simulink model "pfb_fir_generic_test_sim3"  (R2012b)
settings: Solver=VariableStepDiscrete  StartTime=0.0  StopTime=10.0  RelTol=1e-3
model workspace (MAT data in the model file):
  synci = [0 1 2 3 4 5 6 7 8 9 10 11 ... (589826 elements, 294913x2)]
  din0 = [0 1 2 3 4 5 6 7 8 9 10 11 ... (73730 elements, 36865x2)]
  din1 = [0 1 2 3 4 5 6 7 8 9 10 11 ... (73730 elements, 36865x2)]
  din2 = [0 1 2 3 4 5 6 7 8 9 10 11 ... (73730 elements, 36865x2)]
  din3 = [0 1 2 3 4 5 6 7 8 9 10 11 ... (73730 elements, 36865x2)]
  din4 = [0 1 2 3 4 5 6 7 8 9 10 11 ... (73730 elements, 36865x2)]
  din5 = [0 1 2 3 4 5 6 7 8 9 10 11 ... (73730 elements, 36865x2)]
  din6 = [0 1 2 3 4 5 6 7 8 9 10 11 ... (73730 elements, 36865x2)]
  din7 = [0 1 2 3 4 5 6 7 8 9 10 11 ... (73730 elements, 36865x2)]
libraries: xbsIndex_r4 x5585, casper_library_delays x1
(part 21 of 25)

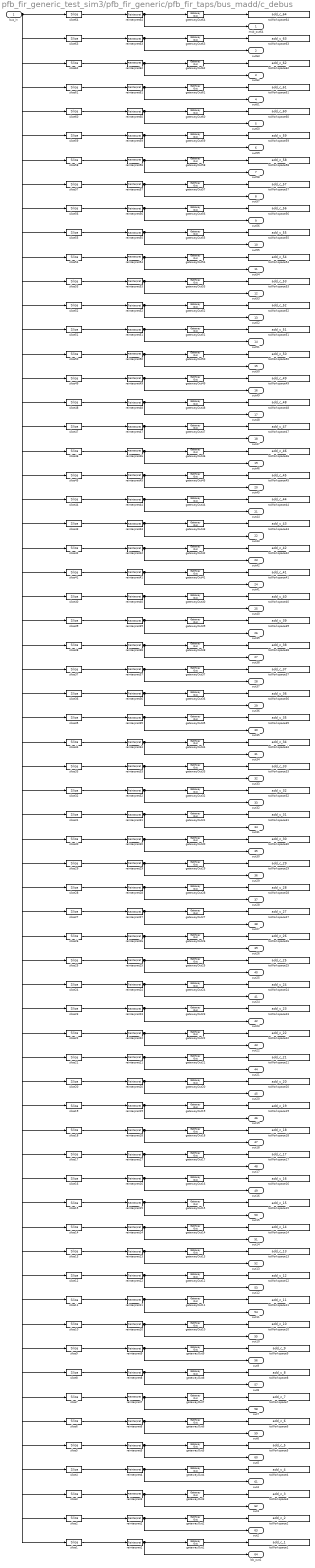
== system pfb_fir_generic_test_sim3/pfb_fir_generic/pfb_fir_taps/bus_madd/c_debus ==
  bus_in : Inport
  gatewayOut{1..64} (64 alike) : xbsIndex_r4/Gateway Out  inherit_from_input=off  hdl_port=off  timing_constraint=None  locs_specified=off  LOCs={}  UseAsDAC=off  DACChannel='1'  block_type=gatewayout
  reinterpret{1..64} (64 alike) : xbsIndex_r4/Reinterpret  force_arith_type=on  arith_type="Signed  (2's comp)"  force_bin_pt=on  bin_pt=26  block_type=reinterpret
  slice1 : xbsIndex_r4/Slice  nbits=30  boolean_output=off  mode=Upper Bit Location + Width  bit1=-1810  base1=MSB of Input  bit0=0  base0=LSB of Input  dbl_ovrd=off  block_type=slice
  slice10 : xbsIndex_r4/Slice  nbits=30  boolean_output=off  mode=Upper Bit Location + Width  bit1=-1540  base1=MSB of Input  bit0=0  base0=LSB of Input  dbl_ovrd=off  block_type=slice
  slice11 : xbsIndex_r4/Slice  nbits=30  boolean_output=off  mode=Upper Bit Location + Width  bit1=-1510  base1=MSB of Input  bit0=0  base0=LSB of Input  dbl_ovrd=off  block_type=slice
  slice12 : xbsIndex_r4/Slice  nbits=30  boolean_output=off  mode=Upper Bit Location + Width  bit1=-1480  base1=MSB of Input  bit0=0  base0=LSB of Input  dbl_ovrd=off  block_type=slice
  slice13 : xbsIndex_r4/Slice  nbits=30  boolean_output=off  mode=Upper Bit Location + Width  bit1=-1450  base1=MSB of Input  bit0=0  base0=LSB of Input  dbl_ovrd=off  block_type=slice
  slice14 : xbsIndex_r4/Slice  nbits=30  boolean_output=off  mode=Upper Bit Location + Width  bit1=-1420  base1=MSB of Input  bit0=0  base0=LSB of Input  dbl_ovrd=off  block_type=slice
  slice15 : xbsIndex_r4/Slice  nbits=30  boolean_output=off  mode=Upper Bit Location + Width  bit1=-1390  base1=MSB of Input  bit0=0  base0=LSB of Input  dbl_ovrd=off  block_type=slice
  slice16 : xbsIndex_r4/Slice  nbits=30  boolean_output=off  mode=Upper Bit Location + Width  bit1=-1360  base1=MSB of Input  bit0=0  base0=LSB of Input  dbl_ovrd=off  block_type=slice
  slice17 : xbsIndex_r4/Slice  nbits=29  boolean_output=off  mode=Upper Bit Location + Width  bit1=-1331  base1=MSB of Input  bit0=0  base0=LSB of Input  dbl_ovrd=off  block_type=slice
  slice18 : xbsIndex_r4/Slice  nbits=29  boolean_output=off  mode=Upper Bit Location + Width  bit1=-1302  base1=MSB of Input  bit0=0  base0=LSB of Input  dbl_ovrd=off  block_type=slice
  slice19 : xbsIndex_r4/Slice  nbits=29  boolean_output=off  mode=Upper Bit Location + Width  bit1=-1273  base1=MSB of Input  bit0=0  base0=LSB of Input  dbl_ovrd=off  block_type=slice
  slice2 : xbsIndex_r4/Slice  nbits=30  boolean_output=off  mode=Upper Bit Location + Width  bit1=-1780  base1=MSB of Input  bit0=0  base0=LSB of Input  dbl_ovrd=off  block_type=slice
  slice20 : xbsIndex_r4/Slice  nbits=29  boolean_output=off  mode=Upper Bit Location + Width  bit1=-1244  base1=MSB of Input  bit0=0  base0=LSB of Input  dbl_ovrd=off  block_type=slice
  slice21 : xbsIndex_r4/Slice  nbits=29  boolean_output=off  mode=Upper Bit Location + Width  bit1=-1215  base1=MSB of Input  bit0=0  base0=LSB of Input  dbl_ovrd=off  block_type=slice
  slice22 : xbsIndex_r4/Slice  nbits=29  boolean_output=off  mode=Upper Bit Location + Width  bit1=-1186  base1=MSB of Input  bit0=0  base0=LSB of Input  dbl_ovrd=off  block_type=slice
  slice23 : xbsIndex_r4/Slice  nbits=29  boolean_output=off  mode=Upper Bit Location + Width  bit1=-1157  base1=MSB of Input  bit0=0  base0=LSB of Input  dbl_ovrd=off  block_type=slice
  slice24 : xbsIndex_r4/Slice  nbits=29  boolean_output=off  mode=Upper Bit Location + Width  bit1=-1128  base1=MSB of Input  bit0=0  base0=LSB of Input  dbl_ovrd=off  block_type=slice
  slice25 : xbsIndex_r4/Slice  nbits=29  boolean_output=off  mode=Upper Bit Location + Width  bit1=-1099  base1=MSB of Input  bit0=0  base0=LSB of Input  dbl_ovrd=off  block_type=slice
  slice26 : xbsIndex_r4/Slice  nbits=29  boolean_output=off  mode=Upper Bit Location + Width  bit1=-1070  base1=MSB of Input  bit0=0  base0=LSB of Input  dbl_ovrd=off  block_type=slice
  slice27 : xbsIndex_r4/Slice  nbits=29  boolean_output=off  mode=Upper Bit Location + Width  bit1=-1041  base1=MSB of Input  bit0=0  base0=LSB of Input  dbl_ovrd=off  block_type=slice
  slice28 : xbsIndex_r4/Slice  nbits=29  boolean_output=off  mode=Upper Bit Location + Width  bit1=-1012  base1=MSB of Input  bit0=0  base0=LSB of Input  dbl_ovrd=off  block_type=slice
  slice29 : xbsIndex_r4/Slice  nbits=29  boolean_output=off  mode=Upper Bit Location + Width  bit1=-983  base1=MSB of Input  bit0=0  base0=LSB of Input  dbl_ovrd=off  block_type=slice
  slice3 : xbsIndex_r4/Slice  nbits=30  boolean_output=off  mode=Upper Bit Location + Width  bit1=-1750  base1=MSB of Input  bit0=0  base0=LSB of Input  dbl_ovrd=off  block_type=slice
  slice30 : xbsIndex_r4/Slice  nbits=29  boolean_output=off  mode=Upper Bit Location + Width  bit1=-954  base1=MSB of Input  bit0=0  base0=LSB of Input  dbl_ovrd=off  block_type=slice
  slice31 : xbsIndex_r4/Slice  nbits=29  boolean_output=off  mode=Upper Bit Location + Width  bit1=-925  base1=MSB of Input  bit0=0  base0=LSB of Input  dbl_ovrd=off  block_type=slice
  slice32 : xbsIndex_r4/Slice  nbits=29  boolean_output=off  mode=Upper Bit Location + Width  bit1=-896  base1=MSB of Input  bit0=0  base0=LSB of Input  dbl_ovrd=off  block_type=slice
  slice33 : xbsIndex_r4/Slice  nbits=28  boolean_output=off  mode=Upper Bit Location + Width  bit1=-868  base1=MSB of Input  bit0=0  base0=LSB of Input  dbl_ovrd=off  block_type=slice
  slice34 : xbsIndex_r4/Slice  nbits=28  boolean_output=off  mode=Upper Bit Location + Width  bit1=-840  base1=MSB of Input  bit0=0  base0=LSB of Input  dbl_ovrd=off  block_type=slice
  slice35 : xbsIndex_r4/Slice  nbits=28  boolean_output=off  mode=Upper Bit Location + Width  bit1=-812  base1=MSB of Input  bit0=0  base0=LSB of Input  dbl_ovrd=off  block_type=slice
  slice36 : xbsIndex_r4/Slice  nbits=28  boolean_output=off  mode=Upper Bit Location + Width  bit1=-784  base1=MSB of Input  bit0=0  base0=LSB of Input  dbl_ovrd=off  block_type=slice
  slice37 : xbsIndex_r4/Slice  nbits=28  boolean_output=off  mode=Upper Bit Location + Width  bit1=-756  base1=MSB of Input  bit0=0  base0=LSB of Input  dbl_ovrd=off  block_type=slice
  slice38 : xbsIndex_r4/Slice  nbits=28  boolean_output=off  mode=Upper Bit Location + Width  bit1=-728  base1=MSB of Input  bit0=0  base0=LSB of Input  dbl_ovrd=off  block_type=slice
  slice39 : xbsIndex_r4/Slice  nbits=28  boolean_output=off  mode=Upper Bit Location + Width  bit1=-700  base1=MSB of Input  bit0=0  base0=LSB of Input  dbl_ovrd=off  block_type=slice
  slice4 : xbsIndex_r4/Slice  nbits=30  boolean_output=off  mode=Upper Bit Location + Width  bit1=-1720  base1=MSB of Input  bit0=0  base0=LSB of Input  dbl_ovrd=off  block_type=slice
  slice40 : xbsIndex_r4/Slice  nbits=28  boolean_output=off  mode=Upper Bit Location + Width  bit1=-672  base1=MSB of Input  bit0=0  base0=LSB of Input  dbl_ovrd=off  block_type=slice
  slice41 : xbsIndex_r4/Slice  nbits=28  boolean_output=off  mode=Upper Bit Location + Width  bit1=-644  base1=MSB of Input  bit0=0  base0=LSB of Input  dbl_ovrd=off  block_type=slice
  slice42 : xbsIndex_r4/Slice  nbits=28  boolean_output=off  mode=Upper Bit Location + Width  bit1=-616  base1=MSB of Input  bit0=0  base0=LSB of Input  dbl_ovrd=off  block_type=slice
  slice43 : xbsIndex_r4/Slice  nbits=28  boolean_output=off  mode=Upper Bit Location + Width  bit1=-588  base1=MSB of Input  bit0=0  base0=LSB of Input  dbl_ovrd=off  block_type=slice
  slice44 : xbsIndex_r4/Slice  nbits=28  boolean_output=off  mode=Upper Bit Location + Width  bit1=-560  base1=MSB of Input  bit0=0  base0=LSB of Input  dbl_ovrd=off  block_type=slice
  slice45 : xbsIndex_r4/Slice  nbits=28  boolean_output=off  mode=Upper Bit Location + Width  bit1=-532  base1=MSB of Input  bit0=0  base0=LSB of Input  dbl_ovrd=off  block_type=slice
  slice46 : xbsIndex_r4/Slice  nbits=28  boolean_output=off  mode=Upper Bit Location + Width  bit1=-504  base1=MSB of Input  bit0=0  base0=LSB of Input  dbl_ovrd=off  block_type=slice
  slice47 : xbsIndex_r4/Slice  nbits=28  boolean_output=off  mode=Upper Bit Location + Width  bit1=-476  base1=MSB of Input  bit0=0  base0=LSB of Input  dbl_ovrd=off  block_type=slice
  slice48 : xbsIndex_r4/Slice  nbits=28  boolean_output=off  mode=Upper Bit Location + Width  bit1=-448  base1=MSB of Input  bit0=0  base0=LSB of Input  dbl_ovrd=off  block_type=slice
  slice49 : xbsIndex_r4/Slice  nbits=28  boolean_output=off  mode=Upper Bit Location + Width  bit1=-420  base1=MSB of Input  bit0=0  base0=LSB of Input  dbl_ovrd=off  block_type=slice
  slice5 : xbsIndex_r4/Slice  nbits=30  boolean_output=off  mode=Upper Bit Location + Width  bit1=-1690  base1=MSB of Input  bit0=0  base0=LSB of Input  dbl_ovrd=off  block_type=slice
  slice50 : xbsIndex_r4/Slice  nbits=28  boolean_output=off  mode=Upper Bit Location + Width  bit1=-392  base1=MSB of Input  bit0=0  base0=LSB of Input  dbl_ovrd=off  block_type=slice
  slice51 : xbsIndex_r4/Slice  nbits=28  boolean_output=off  mode=Upper Bit Location + Width  bit1=-364  base1=MSB of Input  bit0=0  base0=LSB of Input  dbl_ovrd=off  block_type=slice
  slice52 : xbsIndex_r4/Slice  nbits=28  boolean_output=off  mode=Upper Bit Location + Width  bit1=-336  base1=MSB of Input  bit0=0  base0=LSB of Input  dbl_ovrd=off  block_type=slice
  slice53 : xbsIndex_r4/Slice  nbits=28  boolean_output=off  mode=Upper Bit Location + Width  bit1=-308  base1=MSB of Input  bit0=0  base0=LSB of Input  dbl_ovrd=off  block_type=slice
  slice54 : xbsIndex_r4/Slice  nbits=28  boolean_output=off  mode=Upper Bit Location + Width  bit1=-280  base1=MSB of Input  bit0=0  base0=LSB of Input  dbl_ovrd=off  block_type=slice
  slice55 : xbsIndex_r4/Slice  nbits=28  boolean_output=off  mode=Upper Bit Location + Width  bit1=-252  base1=MSB of Input  bit0=0  base0=LSB of Input  dbl_ovrd=off  block_type=slice
  slice56 : xbsIndex_r4/Slice  nbits=28  boolean_output=off  mode=Upper Bit Location + Width  bit1=-224  base1=MSB of Input  bit0=0  base0=LSB of Input  dbl_ovrd=off  block_type=slice
  slice57 : xbsIndex_r4/Slice  nbits=28  boolean_output=off  mode=Upper Bit Location + Width  bit1=-196  base1=MSB of Input  bit0=0  base0=LSB of Input  dbl_ovrd=off  block_type=slice
  slice58 : xbsIndex_r4/Slice  nbits=28  boolean_output=off  mode=Upper Bit Location + Width  bit1=-168  base1=MSB of Input  bit0=0  base0=LSB of Input  dbl_ovrd=off  block_type=slice
  slice59 : xbsIndex_r4/Slice  nbits=28  boolean_output=off  mode=Upper Bit Location + Width  bit1=-140  base1=MSB of Input  bit0=0  base0=LSB of Input  dbl_ovrd=off  block_type=slice
  slice6 : xbsIndex_r4/Slice  nbits=30  boolean_output=off  mode=Upper Bit Location + Width  bit1=-1660  base1=MSB of Input  bit0=0  base0=LSB of Input  dbl_ovrd=off  block_type=slice
  slice60 : xbsIndex_r4/Slice  nbits=28  boolean_output=off  mode=Upper Bit Location + Width  bit1=-112  base1=MSB of Input  bit0=0  base0=LSB of Input  dbl_ovrd=off  block_type=slice
  slice61 : xbsIndex_r4/Slice  nbits=28  boolean_output=off  mode=Upper Bit Location + Width  bit1=-84  base1=MSB of Input  bit0=0  base0=LSB of Input  dbl_ovrd=off  block_type=slice
  slice62 : xbsIndex_r4/Slice  nbits=28  boolean_output=off  mode=Upper Bit Location + Width  bit1=-56  base1=MSB of Input  bit0=0  base0=LSB of Input  dbl_ovrd=off  block_type=slice
  slice63 : xbsIndex_r4/Slice  nbits=28  boolean_output=off  mode=Upper Bit Location + Width  bit1=-28  base1=MSB of Input  bit0=0  base0=LSB of Input  dbl_ovrd=off  block_type=slice
  slice64 : xbsIndex_r4/Slice  nbits=28  boolean_output=off  mode=Upper Bit Location + Width  bit1=0  base1=MSB of Input  bit0=0  base0=LSB of Input  dbl_ovrd=off  block_type=slice
  slice7 : xbsIndex_r4/Slice  nbits=30  boolean_output=off  mode=Upper Bit Location + Width  bit1=-1630  base1=MSB of Input  bit0=0  base0=LSB of Input  dbl_ovrd=off  block_type=slice
  slice8 : xbsIndex_r4/Slice  nbits=30  boolean_output=off  mode=Upper Bit Location + Width  bit1=-1600  base1=MSB of Input  bit0=0  base0=LSB of Input  dbl_ovrd=off  block_type=slice
  slice9 : xbsIndex_r4/Slice  nbits=30  boolean_output=off  mode=Upper Bit Location + Width  bit1=-1570  base1=MSB of Input  bit0=0  base0=LSB of Input  dbl_ovrd=off  block_type=slice
  toWorkspace1 : ToWorkspace  VariableName=add_c_1  SampleTime=-1  SaveFormat=Structure With Time
  toWorkspace10 : ToWorkspace  VariableName=add_c_10  SampleTime=-1  SaveFormat=Structure With Time
  toWorkspace11 : ToWorkspace  VariableName=add_c_11  SampleTime=-1  SaveFormat=Structure With Time
  toWorkspace12 : ToWorkspace  VariableName=add_c_12  SampleTime=-1  SaveFormat=Structure With Time
  toWorkspace13 : ToWorkspace  VariableName=add_c_13  SampleTime=-1  SaveFormat=Structure With Time
  toWorkspace14 : ToWorkspace  VariableName=add_c_14  SampleTime=-1  SaveFormat=Structure With Time
  toWorkspace15 : ToWorkspace  VariableName=add_c_15  SampleTime=-1  SaveFormat=Structure With Time
  toWorkspace16 : ToWorkspace  VariableName=add_c_16  SampleTime=-1  SaveFormat=Structure With Time
  toWorkspace17 : ToWorkspace  VariableName=add_c_17  SampleTime=-1  SaveFormat=Structure With Time
  toWorkspace18 : ToWorkspace  VariableName=add_c_18  SampleTime=-1  SaveFormat=Structure With Time
  toWorkspace19 : ToWorkspace  VariableName=add_c_19  SampleTime=-1  SaveFormat=Structure With Time
  toWorkspace2 : ToWorkspace  VariableName=add_c_2  SampleTime=-1  SaveFormat=Structure With Time
  toWorkspace20 : ToWorkspace  VariableName=add_c_20  SampleTime=-1  SaveFormat=Structure With Time
  toWorkspace21 : ToWorkspace  VariableName=add_c_21  SampleTime=-1  SaveFormat=Structure With Time
  toWorkspace22 : ToWorkspace  VariableName=add_c_22  SampleTime=-1  SaveFormat=Structure With Time
  toWorkspace23 : ToWorkspace  VariableName=add_c_23  SampleTime=-1  SaveFormat=Structure With Time
  toWorkspace24 : ToWorkspace  VariableName=add_c_24  SampleTime=-1  SaveFormat=Structure With Time
  toWorkspace25 : ToWorkspace  VariableName=add_c_25  SampleTime=-1  SaveFormat=Structure With Time
  toWorkspace26 : ToWorkspace  VariableName=add_c_26  SampleTime=-1  SaveFormat=Structure With Time
  toWorkspace27 : ToWorkspace  VariableName=add_c_27  SampleTime=-1  SaveFormat=Structure With Time
  toWorkspace28 : ToWorkspace  VariableName=add_c_28  SampleTime=-1  SaveFormat=Structure With Time
  toWorkspace29 : ToWorkspace  VariableName=add_c_29  SampleTime=-1  SaveFormat=Structure With Time
  toWorkspace3 : ToWorkspace  VariableName=add_c_3  SampleTime=-1  SaveFormat=Structure With Time
  toWorkspace30 : ToWorkspace  VariableName=add_c_30  SampleTime=-1  SaveFormat=Structure With Time
  toWorkspace31 : ToWorkspace  VariableName=add_c_31  SampleTime=-1  SaveFormat=Structure With Time
  toWorkspace32 : ToWorkspace  VariableName=add_c_32  SampleTime=-1  SaveFormat=Structure With Time
  toWorkspace33 : ToWorkspace  VariableName=add_c_33  SampleTime=-1  SaveFormat=Structure With Time
  toWorkspace34 : ToWorkspace  VariableName=add_c_34  SampleTime=-1  SaveFormat=Structure With Time
  toWorkspace35 : ToWorkspace  VariableName=add_c_35  SampleTime=-1  SaveFormat=Structure With Time
  toWorkspace36 : ToWorkspace  VariableName=add_c_36  SampleTime=-1  SaveFormat=Structure With Time
  toWorkspace37 : ToWorkspace  VariableName=add_c_37  SampleTime=-1  SaveFormat=Structure With Time
  toWorkspace38 : ToWorkspace  VariableName=add_c_38  SampleTime=-1  SaveFormat=Structure With Time
  toWorkspace39 : ToWorkspace  VariableName=add_c_39  SampleTime=-1  SaveFormat=Structure With Time
  toWorkspace4 : ToWorkspace  VariableName=add_c_4  SampleTime=-1  SaveFormat=Structure With Time
  toWorkspace40 : ToWorkspace  VariableName=add_c_40  SampleTime=-1  SaveFormat=Structure With Time
  toWorkspace41 : ToWorkspace  VariableName=add_c_41  SampleTime=-1  SaveFormat=Structure With Time
  toWorkspace42 : ToWorkspace  VariableName=add_c_42  SampleTime=-1  SaveFormat=Structure With Time
  toWorkspace43 : ToWorkspace  VariableName=add_c_43  SampleTime=-1  SaveFormat=Structure With Time
  toWorkspace44 : ToWorkspace  VariableName=add_c_44  SampleTime=-1  SaveFormat=Structure With Time
  toWorkspace45 : ToWorkspace  VariableName=add_c_45  SampleTime=-1  SaveFormat=Structure With Time
  toWorkspace46 : ToWorkspace  VariableName=add_c_46  SampleTime=-1  SaveFormat=Structure With Time
  toWorkspace47 : ToWorkspace  VariableName=add_c_47  SampleTime=-1  SaveFormat=Structure With Time
  toWorkspace48 : ToWorkspace  VariableName=add_c_48  SampleTime=-1  SaveFormat=Structure With Time
  toWorkspace49 : ToWorkspace  VariableName=add_c_49  SampleTime=-1  SaveFormat=Structure With Time
  toWorkspace5 : ToWorkspace  VariableName=add_c_5  SampleTime=-1  SaveFormat=Structure With Time
  toWorkspace50 : ToWorkspace  VariableName=add_c_50  SampleTime=-1  SaveFormat=Structure With Time
  toWorkspace51 : ToWorkspace  VariableName=add_c_51  SampleTime=-1  SaveFormat=Structure With Time
  toWorkspace52 : ToWorkspace  VariableName=add_c_52  SampleTime=-1  SaveFormat=Structure With Time
  toWorkspace53 : ToWorkspace  VariableName=add_c_53  SampleTime=-1  SaveFormat=Structure With Time
  toWorkspace54 : ToWorkspace  VariableName=add_c_54  SampleTime=-1  SaveFormat=Structure With Time
  toWorkspace55 : ToWorkspace  VariableName=add_c_55  SampleTime=-1  SaveFormat=Structure With Time
  toWorkspace56 : ToWorkspace  VariableName=add_c_56  SampleTime=-1  SaveFormat=Structure With Time
  toWorkspace57 : ToWorkspace  VariableName=add_c_57  SampleTime=-1  SaveFormat=Structure With Time
  toWorkspace58 : ToWorkspace  VariableName=add_c_58  SampleTime=-1  SaveFormat=Structure With Time
  toWorkspace59 : ToWorkspace  VariableName=add_c_59  SampleTime=-1  SaveFormat=Structure With Time
  toWorkspace6 : ToWorkspace  VariableName=add_c_6  SampleTime=-1  SaveFormat=Structure With Time
  toWorkspace60 : ToWorkspace  VariableName=add_c_60  SampleTime=-1  SaveFormat=Structure With Time
  toWorkspace61 : ToWorkspace  VariableName=add_c_61  SampleTime=-1  SaveFormat=Structure With Time
  toWorkspace62 : ToWorkspace  VariableName=add_c_62  SampleTime=-1  SaveFormat=Structure With Time
  toWorkspace63 : ToWorkspace  VariableName=add_c_63  SampleTime=-1  SaveFormat=Structure With Time
  toWorkspace64 : ToWorkspace  VariableName=add_c_64  SampleTime=-1  SaveFormat=Structure With Time
  toWorkspace7 : ToWorkspace  VariableName=add_c_7  SampleTime=-1  SaveFormat=Structure With Time
  toWorkspace8 : ToWorkspace  VariableName=add_c_8  SampleTime=-1  SaveFormat=Structure With Time
  toWorkspace9 : ToWorkspace  VariableName=add_c_9  SampleTime=-1  SaveFormat=Structure With Time
  msb_out64 : Outport
  out63 : Outport  Port=2
  out62 : Outport  Port=3
  out61 : Outport  Port=4
  out60 : Outport  Port=5
  out59 : Outport  Port=6
  out58 : Outport  Port=7
  out57 : Outport  Port=8
  out56 : Outport  Port=9
  out55 : Outport  Port=10
  out54 : Outport  Port=11
  out53 : Outport  Port=12
  out52 : Outport  Port=13
  out51 : Outport  Port=14
  out50 : Outport  Port=15
  out49 : Outport  Port=16
  out48 : Outport  Port=17
  out47 : Outport  Port=18
  out46 : Outport  Port=19
  out45 : Outport  Port=20
  out44 : Outport  Port=21
  out43 : Outport  Port=22
  out42 : Outport  Port=23
  out41 : Outport  Port=24
  out40 : Outport  Port=25
  out39 : Outport  Port=26
  out38 : Outport  Port=27
  out37 : Outport  Port=28
  out36 : Outport  Port=29
  out35 : Outport  Port=30
  out34 : Outport  Port=31
  out33 : Outport  Port=32
  out32 : Outport  Port=33
  out31 : Outport  Port=34
  out30 : Outport  Port=35
  out29 : Outport  Port=36
  out28 : Outport  Port=37
  out27 : Outport  Port=38
  out26 : Outport  Port=39
  out25 : Outport  Port=40
  out24 : Outport  Port=41
  out23 : Outport  Port=42
  out22 : Outport  Port=43
  out21 : Outport  Port=44
  out20 : Outport  Port=45
  out19 : Outport  Port=46
  out18 : Outport  Port=47
  out17 : Outport  Port=48
  out16 : Outport  Port=49
  out15 : Outport  Port=50
  out14 : Outport  Port=51
  out13 : Outport  Port=52
  out12 : Outport  Port=53
  out11 : Outport  Port=54
  out10 : Outport  Port=55
  out9 : Outport  Port=56
  out8 : Outport  Port=57
  out7 : Outport  Port=58
  out6 : Outport  Port=59
  out5 : Outport  Port=60
  out4 : Outport  Port=61
  out3 : Outport  Port=62
  out2 : Outport  Port=63
  lsb_out1 : Outport  Port=64
  wires:
  bus_in/1 -> slice64/1, slice63/1, slice62/1, slice61/1, slice60/1, slice59/1, slice58/1, slice57/1, slice56/1, slice55/1, slice54/1, slice53/1, slice52/1, slice51/1, slice50/1, slice49/1, slice48/1, slice47/1, slice46/1, slice45/1, slice44/1, slice43/1, slice42/1, slice41/1, slice40/1, slice39/1, slice38/1, slice37/1, slice36/1, slice35/1, slice34/1, slice33/1, slice32/1, slice31/1, slice30/1, slice29/1, slice28/1, slice27/1, slice26/1, slice25/1, slice24/1, slice23/1, slice22/1, slice21/1, slice20/1, slice19/1, slice18/1, slice17/1, slice16/1, slice15/1, slice14/1, slice13/1, slice12/1, slice11/1, slice10/1, slice9/1, slice8/1, slice7/1, slice6/1, slice5/1, slice4/1, slice3/1, slice2/1, slice1/1
  slice64/1 -> reinterpret64/1
  reinterpret64/1 -> gatewayOut64/1, msb_out64/1
  gatewayOut64/1 -> toWorkspace64/1
  slice63/1 -> reinterpret63/1
  reinterpret63/1 -> gatewayOut63/1, out63/1
  gatewayOut63/1 -> toWorkspace63/1
  slice62/1 -> reinterpret62/1
  reinterpret62/1 -> gatewayOut62/1, out62/1
  gatewayOut62/1 -> toWorkspace62/1
  slice61/1 -> reinterpret61/1
  reinterpret61/1 -> gatewayOut61/1, out61/1
  gatewayOut61/1 -> toWorkspace61/1
  slice60/1 -> reinterpret60/1
  reinterpret60/1 -> gatewayOut60/1, out60/1
  gatewayOut60/1 -> toWorkspace60/1
  slice59/1 -> reinterpret59/1
  reinterpret59/1 -> gatewayOut59/1, out59/1
  gatewayOut59/1 -> toWorkspace59/1
  slice58/1 -> reinterpret58/1
  reinterpret58/1 -> gatewayOut58/1, out58/1
  gatewayOut58/1 -> toWorkspace58/1
  slice57/1 -> reinterpret57/1
  reinterpret57/1 -> gatewayOut57/1, out57/1
  gatewayOut57/1 -> toWorkspace57/1
  slice56/1 -> reinterpret56/1
  reinterpret56/1 -> gatewayOut56/1, out56/1
  gatewayOut56/1 -> toWorkspace56/1
  slice55/1 -> reinterpret55/1
  reinterpret55/1 -> gatewayOut55/1, out55/1
  gatewayOut55/1 -> toWorkspace55/1
  slice54/1 -> reinterpret54/1
  reinterpret54/1 -> gatewayOut54/1, out54/1
  gatewayOut54/1 -> toWorkspace54/1
  slice53/1 -> reinterpret53/1
  reinterpret53/1 -> gatewayOut53/1, out53/1
  gatewayOut53/1 -> toWorkspace53/1
  slice52/1 -> reinterpret52/1
  reinterpret52/1 -> gatewayOut52/1, out52/1
  gatewayOut52/1 -> toWorkspace52/1
  slice51/1 -> reinterpret51/1
  reinterpret51/1 -> gatewayOut51/1, out51/1
  gatewayOut51/1 -> toWorkspace51/1
  slice50/1 -> reinterpret50/1
  reinterpret50/1 -> gatewayOut50/1, out50/1
  gatewayOut50/1 -> toWorkspace50/1
  slice49/1 -> reinterpret49/1
  reinterpret49/1 -> gatewayOut49/1, out49/1
  gatewayOut49/1 -> toWorkspace49/1
  slice48/1 -> reinterpret48/1
  reinterpret48/1 -> gatewayOut48/1, out48/1
  gatewayOut48/1 -> toWorkspace48/1
  slice47/1 -> reinterpret47/1
  reinterpret47/1 -> gatewayOut47/1, out47/1
  gatewayOut47/1 -> toWorkspace47/1
  slice46/1 -> reinterpret46/1
  reinterpret46/1 -> gatewayOut46/1, out46/1
  gatewayOut46/1 -> toWorkspace46/1
  slice45/1 -> reinterpret45/1
  reinterpret45/1 -> gatewayOut45/1, out45/1
  gatewayOut45/1 -> toWorkspace45/1
  slice44/1 -> reinterpret44/1
  reinterpret44/1 -> gatewayOut44/1, out44/1
  gatewayOut44/1 -> toWorkspace44/1
  slice43/1 -> reinterpret43/1
  reinterpret43/1 -> gatewayOut43/1, out43/1
  gatewayOut43/1 -> toWorkspace43/1
  slice42/1 -> reinterpret42/1
  reinterpret42/1 -> gatewayOut42/1, out42/1
  gatewayOut42/1 -> toWorkspace42/1
  slice41/1 -> reinterpret41/1
  reinterpret41/1 -> gatewayOut41/1, out41/1
  gatewayOut41/1 -> toWorkspace41/1
  slice40/1 -> reinterpret40/1
  reinterpret40/1 -> gatewayOut40/1, out40/1
  gatewayOut40/1 -> toWorkspace40/1
  slice39/1 -> reinterpret39/1
  reinterpret39/1 -> gatewayOut39/1, out39/1
  gatewayOut39/1 -> toWorkspace39/1
  slice38/1 -> reinterpret38/1
  reinterpret38/1 -> gatewayOut38/1, out38/1
  gatewayOut38/1 -> toWorkspace38/1
  slice37/1 -> reinterpret37/1
  reinterpret37/1 -> gatewayOut37/1, out37/1
  gatewayOut37/1 -> toWorkspace37/1
  slice36/1 -> reinterpret36/1
  reinterpret36/1 -> gatewayOut36/1, out36/1
  gatewayOut36/1 -> toWorkspace36/1
  slice35/1 -> reinterpret35/1
  reinterpret35/1 -> gatewayOut35/1, out35/1
  gatewayOut35/1 -> toWorkspace35/1
  slice34/1 -> reinterpret34/1
  reinterpret34/1 -> gatewayOut34/1, out34/1
  gatewayOut34/1 -> toWorkspace34/1
  slice33/1 -> reinterpret33/1
  reinterpret33/1 -> gatewayOut33/1, out33/1
  gatewayOut33/1 -> toWorkspace33/1
  slice32/1 -> reinterpret32/1
  reinterpret32/1 -> gatewayOut32/1, out32/1
  gatewayOut32/1 -> toWorkspace32/1
  slice31/1 -> reinterpret31/1
  reinterpret31/1 -> gatewayOut31/1, out31/1
  gatewayOut31/1 -> toWorkspace31/1
  slice30/1 -> reinterpret30/1
  reinterpret30/1 -> gatewayOut30/1, out30/1
  gatewayOut30/1 -> toWorkspace30/1
  slice29/1 -> reinterpret29/1
  reinterpret29/1 -> gatewayOut29/1, out29/1
  gatewayOut29/1 -> toWorkspace29/1
  slice28/1 -> reinterpret28/1
  reinterpret28/1 -> gatewayOut28/1, out28/1
  gatewayOut28/1 -> toWorkspace28/1
  slice27/1 -> reinterpret27/1
  reinterpret27/1 -> gatewayOut27/1, out27/1
  gatewayOut27/1 -> toWorkspace27/1
  slice26/1 -> reinterpret26/1
  reinterpret26/1 -> gatewayOut26/1, out26/1
  gatewayOut26/1 -> toWorkspace26/1
  slice25/1 -> reinterpret25/1
  reinterpret25/1 -> gatewayOut25/1, out25/1
  gatewayOut25/1 -> toWorkspace25/1
  slice24/1 -> reinterpret24/1
  reinterpret24/1 -> gatewayOut24/1, out24/1
  gatewayOut24/1 -> toWorkspace24/1
  slice23/1 -> reinterpret23/1
  reinterpret23/1 -> gatewayOut23/1, out23/1
  gatewayOut23/1 -> toWorkspace23/1
  slice22/1 -> reinterpret22/1
  reinterpret22/1 -> gatewayOut22/1, out22/1
  gatewayOut22/1 -> toWorkspace22/1
  slice21/1 -> reinterpret21/1
  reinterpret21/1 -> gatewayOut21/1, out21/1
  gatewayOut21/1 -> toWorkspace21/1
  slice20/1 -> reinterpret20/1
  reinterpret20/1 -> gatewayOut20/1, out20/1
  gatewayOut20/1 -> toWorkspace20/1
  slice19/1 -> reinterpret19/1
  reinterpret19/1 -> gatewayOut19/1, out19/1
  gatewayOut19/1 -> toWorkspace19/1
  slice18/1 -> reinterpret18/1
  reinterpret18/1 -> gatewayOut18/1, out18/1
  gatewayOut18/1 -> toWorkspace18/1
  slice17/1 -> reinterpret17/1
  reinterpret17/1 -> gatewayOut17/1, out17/1
  gatewayOut17/1 -> toWorkspace17/1
  slice16/1 -> reinterpret16/1
  reinterpret16/1 -> gatewayOut16/1, out16/1
  gatewayOut16/1 -> toWorkspace16/1
  slice15/1 -> reinterpret15/1
  reinterpret15/1 -> gatewayOut15/1, out15/1
  gatewayOut15/1 -> toWorkspace15/1
  slice14/1 -> reinterpret14/1
  reinterpret14/1 -> gatewayOut14/1, out14/1
  gatewayOut14/1 -> toWorkspace14/1
  slice13/1 -> reinterpret13/1
  reinterpret13/1 -> gatewayOut13/1, out13/1
  gatewayOut13/1 -> toWorkspace13/1
  slice12/1 -> reinterpret12/1
  reinterpret12/1 -> gatewayOut12/1, out12/1
  gatewayOut12/1 -> toWorkspace12/1
  slice11/1 -> reinterpret11/1
  reinterpret11/1 -> gatewayOut11/1, out11/1
  gatewayOut11/1 -> toWorkspace11/1
  slice10/1 -> reinterpret10/1
  reinterpret10/1 -> gatewayOut10/1, out10/1
  gatewayOut10/1 -> toWorkspace10/1
  slice9/1 -> reinterpret9/1
  reinterpret9/1 -> gatewayOut9/1, out9/1
  gatewayOut9/1 -> toWorkspace9/1
  slice8/1 -> reinterpret8/1
  reinterpret8/1 -> gatewayOut8/1, out8/1
  gatewayOut8/1 -> toWorkspace8/1
  slice7/1 -> reinterpret7/1
  reinterpret7/1 -> gatewayOut7/1, out7/1
  gatewayOut7/1 -> toWorkspace7/1
  slice6/1 -> reinterpret6/1
  reinterpret6/1 -> gatewayOut6/1, out6/1
  gatewayOut6/1 -> toWorkspace6/1
  slice5/1 -> reinterpret5/1
  reinterpret5/1 -> gatewayOut5/1, out5/1
  gatewayOut5/1 -> toWorkspace5/1
  slice4/1 -> reinterpret4/1
  reinterpret4/1 -> gatewayOut4/1, out4/1
  gatewayOut4/1 -> toWorkspace4/1
  slice3/1 -> reinterpret3/1
  reinterpret3/1 -> gatewayOut3/1, out3/1
  gatewayOut3/1 -> toWorkspace3/1
  slice2/1 -> reinterpret2/1
  reinterpret2/1 -> gatewayOut2/1, out2/1
  gatewayOut2/1 -> toWorkspace2/1
  slice1/1 -> reinterpret1/1
  reinterpret1/1 -> gatewayOut1/1, lsb_out1/1
  gatewayOut1/1 -> toWorkspace1/1
